simulink library "Add_Solar_Position"  (R2018b)
settings: Solver=ode45  StartTime=0.0  StopTime=10.0  RelTol=1e-3  EnableMultiTasking=on
undefined symbols (not defined in the file): Azimuth_Angle, Zenith_Angle
libraries: carnot x1
settings Model: Creator=lena.frank  LastModifiedBy=drhf
settings DataIOCC: LimitDataPoints=on  SaveFormat=Array  SignalLoggingSaveFormat=ModelDataLogs
settings OptimizationCC: ExpressionDepthLimit=2147483647  LifeSpan=inf
settings DebuggingCC: UnderspecifiedInitializationDetection=Classic  MergeDetectMultiDrivingBlocksExec=none  SolverPrmCheckMsg=warning  FcnCallInpInsideContextMsg=warning  StateNameClashWarn=warning  SFUnexpectedBacktrackingDiag=warning  SFNoUnconditionalDefaultTransitionDiag=warning  SFExecutionAtInitializationDiag=none
settings HardwareCC: ProdBitPerPointer=32  ProdBitPerSizeT=32  ProdBitPerPtrDiffT=32  ProdLargestAtomicFloat=None  ProdIntDivRoundTo=Undefined  ProdEndianess=Unspecified  ProdWordSize=32  ProdHWDeviceType=32-bit Generic
settings ModelReferenceCC: PropagateSignalLabelsOutOfModel=off
settings SFSimCC: SimUseLocalCustomCode=off
settings RTWCC: RTWUseLocalCustomCode=off
settings CodeAppCC: StateflowObjectComments=on
settings GRTTargetCC: TargetLangStandard=C89/C90 (ANSI)  GeneratePreprocessorConditionals=Disable all  CombineOutputUpdateFcns=off  GRTInterface=on
settings ConfigComp: CovMetricSettings=dw  CovHtmlReporting=on  CovSaveCumulativeToWorkspaceVar=on  CovSaveSingleToWorkspaceVar=on  CovExternalEMLEnable=off

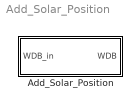
== system Add_Solar_Position ==
  Add_Solar_Position : Subsystem  mask(sun position){longi=-7, lati=50, timezone=-15}
      mask prompts: longi "geographical longitude [degrees] (east negative)"; lati "geographical latitude [degrees] (north positive)"; timezone "longitude of timezone [degrees] (east negative)"
      mask help:
      | This funktion calculates the sun position  and sets it in the weather data vector. Solar zenith angle and azimuth angle (in degrees) (east negative, south = 0°) are set in the weather vector.
      | Timezones:    GMT = 0
      |                       MEZ = -15
      |                       MESZ = -30
      mask init:
      | longi = min(180, max(-180, longi));
      | lati = min(90, max(-90, lati));
      | timezone = min(360, max(-360, timezone));
      mask Help: web(fullfile(path_carnot('help'),'Solar_Position.html'),'-helpbrowser')

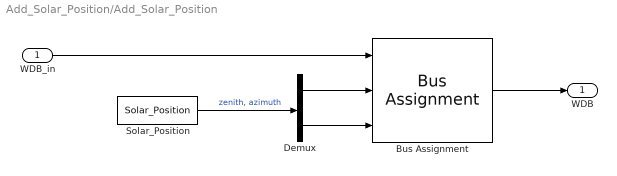
== system Add_Solar_Position/Add_Solar_Position ==
  WDB_in : Inport
  Bus Assignment : BusAssignment  AssignedSignals=Zenith_Angle,Azimuth_Angle
  Demux : Demux  Outputs=2
  Solar_Position : carnot/Basic/Weather_and_Sun/Solar_Position  lati=lati  longi=longi  timezone=timezone
      settings: SourceProductName=Carnot
  WDB : Outport
  wires:
  Solar_Position/1 -> Demux/1  "zenith, azimuth"
  WDB_in/1 -> Bus Assignment/1
  Demux/1 -> Bus Assignment/2
  Demux/2 -> Bus Assignment/3
  Bus Assignment/1 -> WDB/1
